simulink model "HMI_C_S_28379D_FW"  (R2024b)
settings: Solver=ode4  StartTime=0.0  StopTime=Inf  FixedStep=Ts  RelTol=1e-3  EnableMultiTasking=on
InitFcn:
  | Ts=1e-4
model workspace (MAT data in the model file):
  encoderResolution = 2000
  hallOffset = '0.5'
  indexOffset = 850
  polePairs = '4'
libraries: simulink x4, c2837xDlib x2, c280xlib x2, c2802xlib x1
(part 1 of 2)
settings Model: ExtModeTrigDuration=8  Creator=matti  LastModifiedBy=Administrator
settings SolverCC: AlgebraicLoopSolver=TrustRegion  AutoInsertRateTranBlk=on
settings DataIOCC: LimitDataPoints=on  SaveFormat=Array  SignalLoggingSaveFormat=ModelDataLogs  SaveOutput=off  SaveTime=off  ReturnWorkspaceOutputs=off
settings OptimizationCC: DefaultUnderspecifiedDataType=single  OptimizeBlockIOStorage=off  BufferReuse=off  GlobalBufferReuse=off  ExpressionFolding=off  ExpressionDepthLimit=2147483647  LocalBlockOutputs=off  InitFltsAndDblsToZero=on  NoFixptDivByZeroProtection=on  EfficientFloat2IntCast=on  EfficientMapNaN2IntZero=off  LifeSpan=Inf  MaxStackSize=1024  OptimizeDataStoreBuffers=off  BusAssignmentInplaceUpdate=off  EfficientTunableParamExpr=on
settings DebuggingCC: ReadBeforeWriteMsg=DisableAll  WriteAfterWriteMsg=DisableAll  WriteAfterReadMsg=DisableAll  CheckSSInitialOutputMsg=off  UnderspecifiedInitializationDetection=Classic  MergeDetectMultiDrivingBlocksExec=none  SignalResolutionControl=TryResolveAllWithWarning  SolverPrmCheckMsg=warning  InheritedTsInSrcMsg=none  MultiTaskDSMMsg=none  MultiTaskCondExecSysMsg=none  TasksWithSamePriorityMsg=none  SigSpecEnsureSampleTimeMsg=none  IntegerOverflowMsg=none  ParameterPrecisionLossMsg=none  FcnCallInpInsideContextMsg=warning  UnconnectedInputMsg=warning  UnconnectedOutputMsg=warning  UnconnectedLineMsg=warning  StateNameClashWarn=warning  SFUnexpectedBacktrackingDiag=warning  SFNoUnconditionalDefaultTransitionDiag=warning  SFExecutionAtInitializationDiag=none  IntegerSaturationMsg=none  ArithmeticOperatorsInVariantConditions=warning
settings HardwareCC: ProdBitPerChar=16  ProdBitPerInt=16  ProdBitPerPointer=32  ProdBitPerSizeT=32  ProdBitPerPtrDiffT=32  ProdLargestAtomicInteger=Integer  ProdLargestAtomicFloat=None  ProdWordSize=16  ProdLongLongMode=on  ProdHWDeviceType=Texas Instruments->C2000  TargetBitPerChar=16  TargetBitPerInt=16  TargetBitPerPointer=16  TargetLargestAtomicInteger=Integer  TargetIntDivRoundTo=Zero  TargetEndianess=LittleEndian  TargetWordSize=16  TargetHWDeviceType=TI C2000  HardwareBoardFeatureSet=SoCBlockset
settings ModelReferenceCC: EnableRefExpFcnMdlSchedulingChecks=on  PropagateSignalLabelsOutOfModel=off
settings SFSimCC: SimUseLocalCustomCode=off  MATLABDynamicMemAlloc=off  CustomCodeUndefinedFunction=UseInterfaceOnly
settings RTWCC: Description=Embedded Coder  SystemTargetFile=ert.tlc  HardwareBoard=TI Delfino F28379D LaunchPad  TemplateMakefile=ert_default_tmf  GenerateReport=on  RTWUseLocalCustomCode=off  Toolchain=Texas Instruments Code Composer Studio (C2000)  IncludeHyperlinkInReport=on  LaunchReport=on  CodeProfilingSaveOptions=MetricsOnly  GenerateTraceInfo=on  GenerateTraceReport=on  GenerateTraceReportSl=on  GenerateTraceReportSf=on  GenerateTraceReportEml=on  GPUComputeCapability=3.5
settings CodeAppCC: IgnoreCustomStorageClasses=off  CustomSymbolStrType=$N$R$M  StateflowObjectComments=on  InternalIdentifier=Classic
settings ERTTargetCC: CodeReplacementLibrary=TI C28x  MultiwordLength=2048  SupportContinuousTime=on  ExtModeTransport=4  ExtModeStaticAlloc=on  ExtModeAutomaticAllocSize=off  ExtModeStaticAllocSize=10000  ExtModeMexFile=ext_xcp  ExtModeIntrfLevel=Level2 - Open  InlinedParameterPlacement=Hierarchical  ConvertIfToSwitch=off  SuppressUnreachableDefaultCases=off  MemSecPackage=tic2000demospkg  MemSecFuncExecute=code_ramfuncs  DynamicArrayContainerType=coder::array
settings ConfigComp: CovMetricSettings=dw  CovSaveCumulativeToWorkspaceVar=on  CovSaveSingleToWorkspaceVar=on  CovExternalEMLEnable=off  CovSFcnEnable=off
settings SimscapeCC: SimscapeNormalizeSystem=off

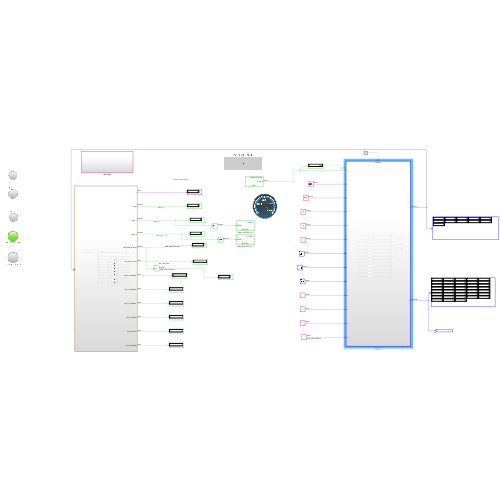
[thumbnail: Simulink's stored preview of the top-level diagram]
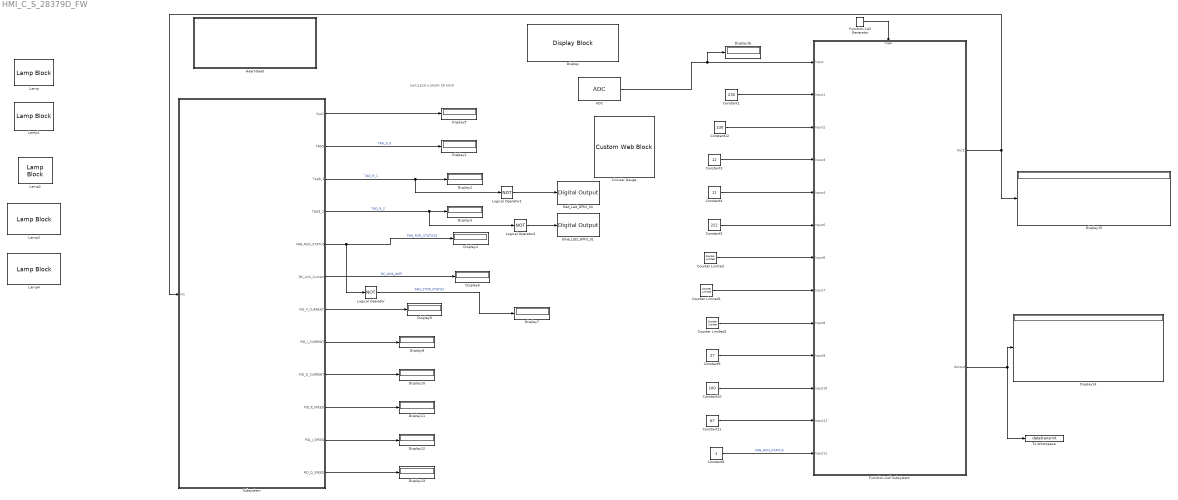
== system HMI_C_S_28379D_FW ==
  note: SHAILESH KUMAR SR MGR
  ADC : c2802xlib/ADC  blkParamProc=C2000_Type4  ADCModule=D  samplingMode=Single sample mode  ADCResolution=12-bit (Single-ended input)  useSOC1=SOC0  useSOC2=SOC0_SOC1  SOCAcquisitionWindow=15  SOCTriggerSource=Software  SOCInterruptTrigger=No ADCINT  Ts=0.001  dType=uint16  postInterrupt=off  interruptSel=ADCINT1  ADCINTContinuous=on  endma=off  chdma=1  conv1=ADCINA0  conv2=ADCINA0 and ADCINB0  conv1_Type4=ADCIN14  conv2_Type4=ADCIN0 and ADCIN1
      settings: LibrarySourceBlock=c2837xDlib/ADC
  Blue_LED_GPIO_31 : c2837xDlib/Digital Output  GPIO_Number=GPIO24~GPIO31  GPIO_Bit0=off  GPIO_BIT0_Toggle=off  GPIO_Bit1=off  GPIO_BIT1_Toggle=off  GPIO_Bit2=off  GPIO_BIT2_Toggle=off  GPIO_Bit3=off  GPIO_BIT3_Toggle=off  GPIO_Bit4=off  GPIO_BIT4_Toggle=off  GPIO_Bit5=off  GPIO_BIT5_Toggle=off  GPIO_Bit6=off  GPIO_BIT6_Toggle=off  GPIO_Bit7=on  GPIO_BIT7_Toggle=off
  Circular Gauge : CustomWebBlock  LabelPosition=Hide  ShowInitialText=on  Configuration="{\"components\":[{\"name\":\"CircularScaleComponent\",\"settings\":{\"bounds\":{\"max\":4096,\"min\":0,\"tickInterval\":\"auto\"},\"direction\":\"cw\",\"flipLimits\":0,\"innerRadius\":0.75,\"internalTickHeightScaleFactor\":1,\"labelColor\":[255,255,200],\"labelFont\":{\"font\":\"Arial\",\"fontSize\":12},\"labelRadius\":0.528,\"labelTransparency\":1,\"minorTickHeightScaleFactor\":0.2,\"needleImage\":{\"size\":[200,50],\"src\":\"data:image\\/svg+xml;base64,PD94bWwgdmVyc2lvbj0iMS4wIiBlbmNvZGluZz0idXRmLTgiPz4KPCEtLSBHZW5lcmF0b3I6IEFkb2JlIElsbHVzdHJhdG9yIDI0LjEuMiwgU1ZHIEV4cG9ydCBQbHVnLUluIC4gU1ZHIFZlcnNpb246IDYuMDAgQnVpbGQgMCkgIC0tPgo8c3ZnIHZlcnNpb249IjEuMSIgaWQ9IkxheWVyXzEiIHhtbG5zPSJodHRwOi8vd3d3LnczLm9yZy8yMDAwL3N2ZyIgeG1sbnM6eGxpbms9Imh0dHA6Ly93d3cudzMub3JnLzE5OTkveGxpbmsiIHg9IjBweCIgeT0iMHB4IgoJIHZpZXdCb3g9IjAgMCAyMDAgNTAiIHN0eWxlPSJlbmFibGUtYmFja2dyb3VuZDpuZXcgMCAwIDIwMCA1MDsiIHhtbDpzcGFjZT0icHJlc2VydmUiPgo8c3R5bGUgdHlwZT0idGV4dC9jc3MiPgoJLnN0MHtmaWxsOiNFQzIxMjc7fQo8L3N0eWxlPgo8cGF0aCBjbGFzcz0ic3QwIiBkPSJNMTYyLjgsMTMuN0MxNjksNC40LDE4MS43LDEuOSwxOTEsOC4xczExLjgsMTguOSw1LjYsMjguMnMtMTguOSwxMS44LTI4LjIsNS42bDAsMAoJQzE1OS4xLDM1LjYsMTU2LjYsMjMsMTYyLjgsMTMuN0wxNjIuOCwxMy43eiBNMTY1LjgsMTUuOGMtNS4xLDcuNi0zLjEsMTcuOSw0LjYsMjNjNy42LDUuMSwxNy45LDMuMSwyMy00LjYKCWM1LjEtNy42LDMuMS0xNy45LTQuNi0yM2wwLDBDMTgxLjIsNi4yLDE3MC45LDguMiwxNjUuOCwxNS44eiIvPgo8cGF0aCBjbGFzcz0ic3QwIiBkPSJNMC40LDI1Ljl2LTMuM2wxNTktMi41Yy0wLjcsMi42LTAuNyw1LjIsMCw3LjhMMC40LDI1Ljl6Ii8+CjxjaXJjbGUgY2xhc3M9InN0MCIgY3g9IjE3OS42IiBjeT0iMjQiIHI9IjAuNyIvPgo8L3N2Zz4K\"},\"needleOffset\":[0.18464878250906522,0],\"needleOrientation\":-45,\"needleRotation\":180,\"needleSize\":{\"height\":0.11741692305346914,\"width\":0.46108337545091255},\"outerRadius\":0.9,\"position\":[0.05,0.05,0.9,0.9],\"referencePoint\":\"auto\",\"scaleAngle\":270,\"scaleAngleOffset\":135,\"scaleColors\":[],\"scaleColorsSize\":0.2,\"scaleDirection\":\"CW\",\"scalePosition\":[0,0,1,1],\"showLabels\":1,\"showMinorTicks\":1,\"showSpanLine\":1,\"showTicks\":1,\"tickColor\":[252,252,197],\"tickTransparency\":1,\"valueBarColor\":[0,114,189],\"valueBarPosition\":[0,0,1,1],\"valueBarSize\":0.2,\"valueBarTransparency\":1}},{\"name\":\"BackgroundImageComponent\",\"settings\":{\"image\":{\"size\":[500,500],\"src\":\"data:image\\/svg+xml;base64,PD94bWwgdmVyc2lvbj0iMS4wIiBlbmNvZGluZz0iVVRGLTgiIHN0YW5kYWxvbmU9Im5vIj8+CjxzdmcKICAgeG1sbnM6ZGM9Imh0dHA6Ly9wdXJsLm9yZy9kYy9lbGVtZW50cy8xLjEvIgogICB4bWxuczpjYz0iaHR0cDovL2NyZWF0aXZlY29tbW9ucy5vcmcvbnMjIgogICB4bWxuczpyZGY9Imh0dHA6Ly93d3cudzMub3JnLzE5OTkvMDIvMjItcmRmLXN5bnRheC1ucyMiCiAgIHhtbG5zOnN2Zz0iaHR0cDovL3d3dy53My5vcmcvMjAwMC9zdmciCiAgIHhtbG5zPSJodHRwOi8vd3d3LnczLm9yZy8yMDAwL3N2ZyIKICAgeG1sbnM6 ...(+9964 chars)\"},\"position\":[0,0,1,1],\"scaleMode\":\"0\"}},{\"name\":\"ForegroundImageComponent\",\"settings\":{\"image\":{\"size\":[0,0],\"src\":\"default\",\"srcOrientation\":[]},\"isForeground\":1,\"position\":[0,0,1,1],\"scaleMode\":\"0\"}}],\"settings\":{\"BindingType\":\"signal\",\"aspectRatio\":1.032258064516129,\"backgroundColor\":[0,0,0,\"1\"],\"backgroundOffset\":1,\"backgroundOpacity\":1,\"direction\":\"cw\",\"fixedAspectRatio\":\"on\",\"flipLimits\":0,\"orientation\":\"horizontal\",\"showBackgroundColor\":false,\"value\":0,\"version\":\"R2023a\"},\"type\":\"CircularGauge\"}"
  Constant1 : Constant  Value=230  OutDataTypeStr=uint16
  Constant10 : Constant  Value=100  OutDataTypeStr=uint16
  Constant11 : Constant  Value=67  OutDataTypeStr=uint16
  Constant12 : Constant  Value=230  OutDataTypeStr=uint16
  Constant3 : Constant  Value=12  OutDataTypeStr=uint16
  Constant4 : Constant  Value=11  OutDataTypeStr=uint16
  Constant5 : Constant  Value=222  OutDataTypeStr=uint16
  Constant6 : Constant  OutDataTypeStr=uint8
  Constant9 : Constant  Value=27  OutDataTypeStr=uint16
  Counter Limited : simulink/Sources/Counter Limited  uplimit=999  tsamp=-1
  Counter Limited1 : simulink/Sources/Counter Limited  uplimit=999  tsamp=-1
  Counter Limited2 : simulink/Sources/Counter Limited  uplimit=999  tsamp=-1
  Display : DisplayBlock  Transparency=1
  Display{1..16} (16 alike) : Display
  Function-Call Generator : simulink/Ports & Subsystems/Function-Call Generator  sample_time=0.1  numberOfIterations=1  DisallowWideOutput=off
  Function-Call Subsystem : Subsystem  TreatAsAtomicUnit=on
  Heart-Beat : Subsystem
  Lamp : LampBlock
  Lamp1 : LampBlock
  Lamp2 : LampBlock
  Lamp3 : LampBlock  LabelPosition=Bottom
  Lamp4 : LampBlock  LabelPosition=Bottom
  Logical Operator : Logic  Operator=NOT  AllPortsSameDT=off  OutDataTypeStr=boolean
  Logical Operator1 : Logic  Operator=NOT  AllPortsSameDT=off  OutDataTypeStr=boolean
  Logical Operator2 : Logic  Operator=NOT  AllPortsSameDT=off  OutDataTypeStr=boolean
  Red_Led_GPIO_34 : c2837xDlib/Digital Output  GPIO_Number=GPIO32~GPIO39  GPIO_Bit0=off  GPIO_BIT0_Toggle=off  GPIO_Bit1=off  GPIO_BIT1_Toggle=off  GPIO_Bit2=on  GPIO_BIT2_Toggle=off  GPIO_Bit3=off  GPIO_BIT3_Toggle=off  GPIO_Bit4=off  GPIO_BIT4_Toggle=off  GPIO_Bit5=off  GPIO_BIT5_Toggle=off  GPIO_Bit6=off  GPIO_BIT6_Toggle=off  GPIO_Bit7=off  GPIO_BIT7_Toggle=off
  Subsystem : Subsystem
  To Workspace : ToWorkspace  VariableName=datatransmit  SampleTime=-1
      settings: Save2DSignal=2-D array (concatenate along first dimension)
  wires:
  Subsystem/12(PID_D_SPEED) -> Display13/1
  Subsystem/1(Out1) -> Display5/1
  Subsystem/5(FAN_RUN_STATUS) -> Display4/1, Logical Operator/1  "FAN_RUN_STATUSS"
  Subsystem/4(TAG9_2) -> Logical Operator2/1, Display3/1  "TAG_9_2"
  Subsystem/3(Tag9_1) -> Logical Operator1/1, Display2/1  "TAG_9_1"
  Subsystem/6(DC_Link_Current) -> Display6/1  "DC_LINK_AMP"
  Subsystem/2(TAG9) -> Display1/1  "TAG_9_0"
  Subsystem/10(PID_P_SPEED) -> Display11/1
  Subsystem/9(PID_D_CURRENT) -> Display10/1
  Subsystem/7(PID_P_CURRENT) -> Display9/1
  Subsystem/8(PID_I_CURRENT) -> Display8/1
  Subsystem/11(PID_I_SPEED) -> Display12/1
  Logical Operator/1 -> Display7/1  "FAN_STOP_STATUS"
  Function-Call Generator/1 -> Function-Call Subsystem/Trigger
  Function-Call Subsystem/1(Out2) -> Subsystem/1(In1), Display15/1
  ADC/1 -> Display16/1, Function-Call Subsystem/1(Input)
  Constant1/1 -> Function-Call Subsystem/2(Input1)
  Constant12/1 -> Function-Call Subsystem/3(Input2)
  Constant3/1 -> Function-Call Subsystem/4(Input3)
  Constant4/1 -> Function-Call Subsystem/5(Input4)
  Constant5/1 -> Function-Call Subsystem/6(Input5)
  Counter Limited/1 -> Function-Call Subsystem/7(Input6)
  Counter Limited1/1 -> Function-Call Subsystem/8(Input7)
  Counter Limited2/1 -> Function-Call Subsystem/9(Input8)
  Constant9/1 -> Function-Call Subsystem/10(Input9)
  Constant10/1 -> Function-Call Subsystem/11(Input10)
  Constant11/1 -> Function-Call Subsystem/12(Input11)
  Constant6/1 -> Function-Call Subsystem/13(Input12)  "FAN_RUN_STATUS"
  Function-Call Subsystem/2(Output) -> To Workspace/1, Display14/1
  Logical Operator1/1 -> Red_Led_GPIO_34/1
  Logical Operator2/1 -> Blue_LED_GPIO_31/1

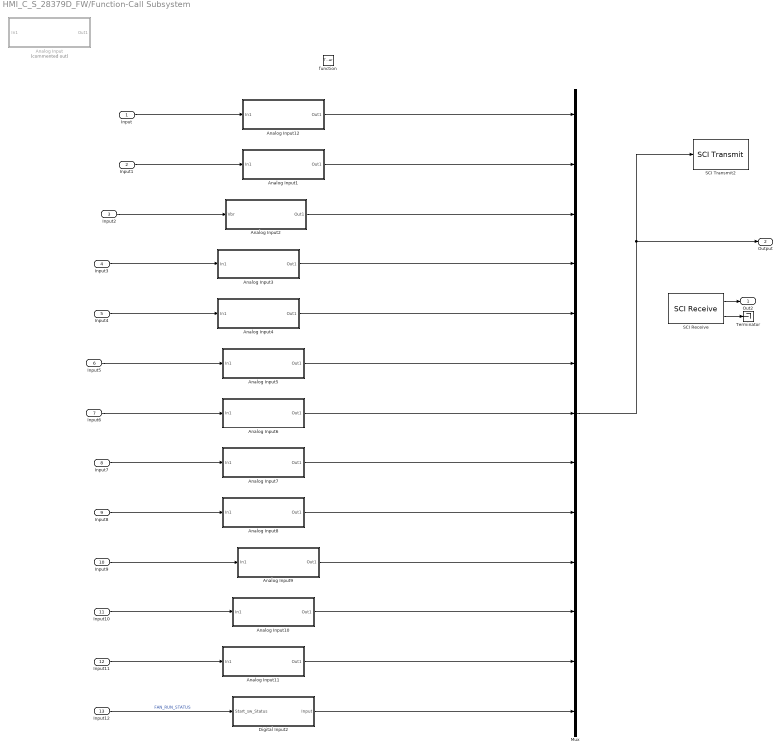
== system HMI_C_S_28379D_FW/Function-Call Subsystem ==
  Input : Inport
  Input1 : Inport  Port=2
  Input2 : Inport  Port=3
  Input3 : Inport  Port=4
  Input4 : Inport  Port=5
  Input5 : Inport  Port=6
  Input6 : Inport  Port=7
  Input7 : Inport  Port=8
  Input8 : Inport  Port=9
  Input9 : Inport  Port=10
  Input10 : Inport  Port=11
  Input11 : Inport  Port=12
  Input12 : Inport  Port=13
  function : TriggerPort  TriggerType=function-call  VariantControl=(inherit)
  Analog Input : Subsystem  Commented=on
  Analog Input1 : Subsystem
  Analog Input10 : Subsystem
  Analog Input11 : Subsystem
  Analog Input12 : Subsystem
  Analog Input2 : Subsystem
  Analog Input3 : Subsystem
  Analog Input4 : Subsystem
  Analog Input5 : Subsystem
  Analog Input6 : Subsystem
  Analog Input7 : Subsystem
  Analog Input8 : Subsystem
  Analog Input9 : Subsystem
  Digital Input2 : Subsystem
  Mux : Mux  Inputs=13
  SCI Receive : c280xlib/SCI Receive  Priority=2  sciModule=B  dataHead='S'  headerCheckMaxCount=16  dataTail='E'  dataType=uint8  dataLenOptions=Length via dialog  dataDim=11  maxDataLength=1  initValue=0  errOption=Output the last received value  errValue=0  sampleTime=-1  blockingMode=off  timeOut=inf  outputStatus=on
      settings: LibrarySourceBlock=c2837xDlib/SCI Receive
  SCI Transmit2 : c280xlib/SCI Transmit  sciModule=B  dataHead='S'  dataTail='E'  frameSize=[1 38]  blockingMode=on  outputStatus=off
      settings: LibrarySourceBlock=c2837xDlib/SCI Transmit
  Terminator : Terminator
  Out2 : Outport
  Output : Outport  Port=2
  wires:
  SCI Receive/1 -> Out2/1
  SCI Receive/2 -> Terminator/1
  Analog Input1/1(Out1) -> Mux/2
  Analog Input2/1(Out1) -> Mux/3
  Analog Input9/1(Out1) -> Mux/10
  Analog Input7/1(Out1) -> Mux/8
  Analog Input4/1(Out1) -> Mux/5
  Analog Input5/1(Out1) -> Mux/6
  Digital Input2/1(Input) -> Mux/13
  Analog Input8/1(Out1) -> Mux/9
  Analog Input10/1(Out1) -> Mux/11
  Analog Input11/1(Out1) -> Mux/12
  Analog Input12/1(Out1) -> Mux/1
  Input1/1 -> Analog Input1/1(In1)
  Input2/1 -> Analog Input2/1(Vbr)
  Input/1 -> Analog Input12/1(In1)
  Input9/1 -> Analog Input9/1(In1)
  Input12/1 -> Digital Input2/1(Start_sw_Status)  "FAN_RUN_STATUS"
  Analog Input3/1(Out1) -> Mux/4
  Input11/1 -> Analog Input11/1(In1)
  Analog Input6/1(Out1) -> Mux/7
  Input10/1 -> Analog Input10/1(In1)
  Mux/1 -> SCI Transmit2/1, Output/1
  Input3/1 -> Analog Input3/1(In1)
  Input4/1 -> Analog Input4/1(In1)
  Input5/1 -> Analog Input5/1(In1)
  Input6/1 -> Analog Input6/1(In1)
  Input7/1 -> Analog Input7/1(In1)
  Input8/1 -> Analog Input8/1(In1)

== system HMI_C_S_28379D_FW/Heart-Beat ==

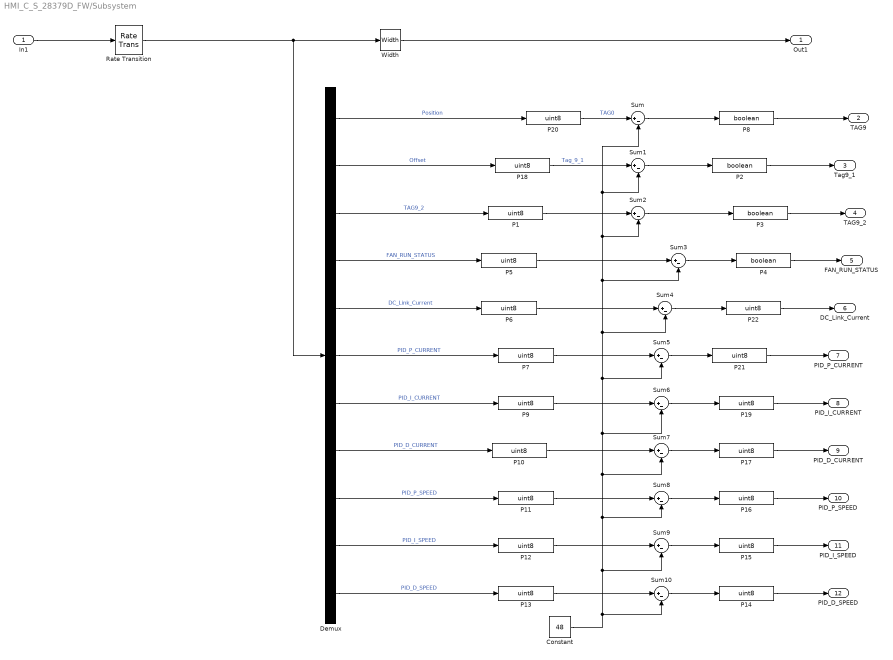
== system HMI_C_S_28379D_FW/Subsystem ==
  In1 : Inport
  Constant : Constant  Value=48  OutDataTypeStr=uint8
  Demux : Demux  Outputs=11
  P{1,5..7,9..22} (18 alike) : DataTypeConversion  OutDataTypeStr=uint8  SaturateOnIntegerOverflow=off  RndMeth=Floor
  P{2..4,8} (4 alike) : DataTypeConversion  OutDataTypeStr=boolean  SaturateOnIntegerOverflow=off  RndMeth=Floor
  Rate Transition : RateTransition
  Sum{,1..10} (11 alike) : Sum  Inputs=|+-
  Width : Width  DataType=uint8
  Out1 : Outport
  TAG9 : Outport  Port=2
  Tag9_1 : Outport  Port=3
  TAG9_2 : Outport  Port=4
  FAN_RUN_STATUS : Outport  Port=5
  DC_Link_Current : Outport  Port=6
  PID_P_CURRENT : Outport  Port=7
  PID_I_CURRENT : Outport  Port=8
  PID_D_CURRENT : Outport  Port=9
  PID_P_SPEED : Outport  Port=10
  PID_I_SPEED : Outport  Port=11
  PID_D_SPEED : Outport  Port=12
  wires:
  Demux/2 -> P18/1  "Offset"
  Demux/1 -> P20/1  "Position"
  Width/1 -> Out1/1
  In1/1 -> Rate Transition/1
  P20/1 -> Sum/1  "TAG0"
  Sum/1 -> P8/1
  P18/1 -> Sum1/1  "Tag_9_1"
  Sum1/1 -> P2/1
  Demux/3 -> P1/1  "TAG9_2"
  Sum2/1 -> P3/1
  Demux/4 -> P5/1  "FAN_RUN_STATUS"
  Sum3/1 -> P4/1
  Demux/5 -> P6/1  "DC_Link_Current"
  Sum4/1 -> P22/1
  Demux/6 -> P7/1  "PID_P_CURRENT"
  Sum5/1 -> P21/1
  Demux/7 -> P9/1  "PID_I_CURRENT"
  Sum6/1 -> P19/1
  Demux/8 -> P10/1  "PID_D_CURRENT"
  Sum7/1 -> P17/1
  Demux/9 -> P11/1  "PID_P_SPEED"
  Sum8/1 -> P16/1
  Demux/10 -> P12/1  "PID_I_SPEED"
  Sum9/1 -> P15/1
  Demux/11 -> P13/1  "PID_D_SPEED"
  Constant/1 -> Sum10/2, Sum9/2, Sum8/2, Sum7/2, Sum6/2, Sum5/2, Sum4/2, Sum3/2, Sum2/2, Sum1/2, Sum/2
  Sum10/1 -> P14/1
  P8/1 -> TAG9/1
  P1/1 -> Sum2/1
  P2/1 -> Tag9_1/1
  P3/1 -> TAG9_2/1
  P4/1 -> FAN_RUN_STATUS/1
  P5/1 -> Sum3/1
  P6/1 -> Sum4/1
  P7/1 -> Sum5/1
  P9/1 -> Sum6/1
  P10/1 -> Sum7/1
  P11/1 -> Sum8/1
  P12/1 -> Sum9/1
  P13/1 -> Sum10/1
  Rate Transition/1 -> Demux/1, Width/1
  P14/1 -> PID_D_SPEED/1
  P15/1 -> PID_I_SPEED/1
  P16/1 -> PID_P_SPEED/1
  P17/1 -> PID_D_CURRENT/1
  P19/1 -> PID_I_CURRENT/1
  P21/1 -> PID_P_CURRENT/1
  P22/1 -> DC_Link_Current/1

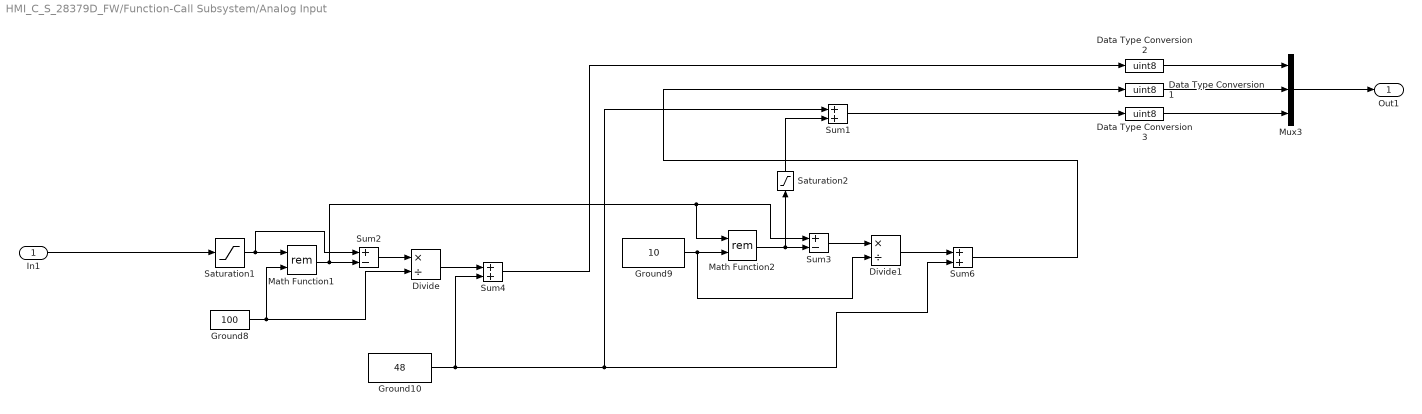
== system HMI_C_S_28379D_FW/Function-Call Subsystem/Analog Input ==
  In1 : Inport
  Data Type Conversion1 : DataTypeConversion  OutDataTypeStr=uint8  SaturateOnIntegerOverflow=off  RndMeth=Floor
  Data Type Conversion2 : DataTypeConversion  OutDataTypeStr=uint8  SaturateOnIntegerOverflow=off  RndMeth=Floor
  Data Type Conversion3 : DataTypeConversion  OutDataTypeStr=uint8  SaturateOnIntegerOverflow=off  RndMeth=Floor
  Divide : Product  Inputs=*/  OutDataTypeStr=int16
  Divide1 : Product  Inputs=*/  OutDataTypeStr=int16
  Ground10 : Constant  Value=48  OutDataTypeStr=int16
  Ground8 : Constant  Value=100  OutDataTypeStr=int16
  Ground9 : Constant  Value=10  OutDataTypeStr=int16
  Math Function1 : Math  Operator=rem  SignedPower=on
  Math Function2 : Math  Operator=rem  SignedPower=on
  Mux3 : Mux  Inputs=3
  Saturation1 : Saturate  UpperLimit=999  LowerLimit=0  OutDataTypeStr=int16
  Saturation2 : Saturate  UpperLimit=9  LowerLimit=0
  Sum1 : Sum  OutDataTypeStr=uint8
  Sum2 : Sum  Inputs=+-  OutDataTypeStr=double
  Sum3 : Sum  Inputs=+-
  Sum4 : Sum  OutDataTypeStr=uint8
  Sum6 : Sum  OutDataTypeStr=uint8
  Out1 : Outport
  wires:
  Saturation1/1 -> Sum2/1, Math Function1/1
  Ground8/1 -> Divide/2, Math Function1/2
  Sum4/1 -> Data Type Conversion2/1
  Sum1/1 -> Data Type Conversion3/1
  Divide/1 -> Sum4/1
  Divide1/1 -> Sum6/1
  Sum2/1 -> Divide/1
  In1/1 -> Saturation1/1
  Data Type Conversion2/1 -> Mux3/1
  Mux3/1 -> Out1/1
  Data Type Conversion3/1 -> Mux3/3
  Data Type Conversion1/1 -> Mux3/2
  Math Function1/1 -> Sum2/2, Math Function2/1, Sum3/1
  Sum3/1 -> Divide1/1
  Sum6/1 -> Data Type Conversion1/1
  Ground10/1 -> Sum4/2, Sum6/2, Sum1/1
  Ground9/1 -> Divide1/2, Math Function2/2
  Math Function2/1 -> Sum3/2, Saturation2/1
  Saturation2/1 -> Sum1/2

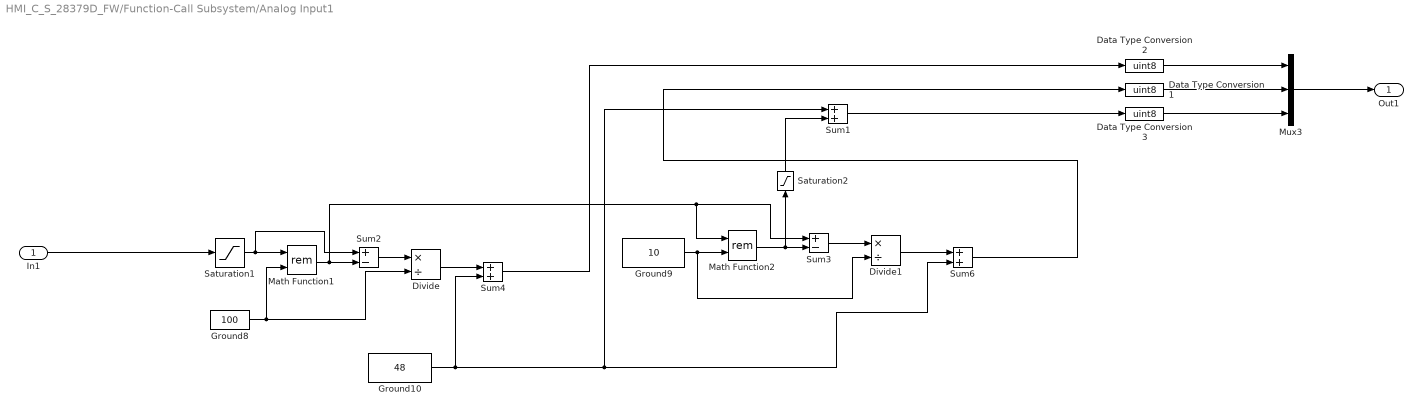
== system HMI_C_S_28379D_FW/Function-Call Subsystem/Analog Input1 ==
  In1 : Inport
  Data Type Conversion1 : DataTypeConversion  OutDataTypeStr=uint8  SaturateOnIntegerOverflow=off  RndMeth=Floor
  Data Type Conversion2 : DataTypeConversion  OutDataTypeStr=uint8  SaturateOnIntegerOverflow=off  RndMeth=Floor
  Data Type Conversion3 : DataTypeConversion  OutDataTypeStr=uint8  SaturateOnIntegerOverflow=off  RndMeth=Floor
  Divide : Product  Inputs=*/  OutDataTypeStr=int16
  Divide1 : Product  Inputs=*/  OutDataTypeStr=int16
  Ground10 : Constant  Value=48  OutDataTypeStr=int16
  Ground8 : Constant  Value=100  OutDataTypeStr=int16
  Ground9 : Constant  Value=10  OutDataTypeStr=int16
  Math Function1 : Math  Operator=rem  SignedPower=on
  Math Function2 : Math  Operator=rem  SignedPower=on
  Mux3 : Mux  Inputs=3
  Saturation1 : Saturate  UpperLimit=999  LowerLimit=0  OutDataTypeStr=int16
  Saturation2 : Saturate  UpperLimit=9  LowerLimit=0
  Sum1 : Sum  OutDataTypeStr=uint8
  Sum2 : Sum  Inputs=+-  OutDataTypeStr=double
  Sum3 : Sum  Inputs=+-
  Sum4 : Sum  OutDataTypeStr=uint8
  Sum6 : Sum  OutDataTypeStr=uint8
  Out1 : Outport
  wires:
  Saturation1/1 -> Sum2/1, Math Function1/1
  Ground8/1 -> Divide/2, Math Function1/2
  Sum4/1 -> Data Type Conversion2/1
  Sum1/1 -> Data Type Conversion3/1
  Divide/1 -> Sum4/1
  Divide1/1 -> Sum6/1
  Sum2/1 -> Divide/1
  In1/1 -> Saturation1/1
  Data Type Conversion2/1 -> Mux3/1
  Mux3/1 -> Out1/1
  Data Type Conversion3/1 -> Mux3/3
  Data Type Conversion1/1 -> Mux3/2
  Math Function1/1 -> Sum2/2, Math Function2/1, Sum3/1
  Sum3/1 -> Divide1/1
  Sum6/1 -> Data Type Conversion1/1
  Ground10/1 -> Sum4/2, Sum6/2, Sum1/1
  Ground9/1 -> Divide1/2, Math Function2/2
  Math Function2/1 -> Sum3/2, Saturation2/1
  Saturation2/1 -> Sum1/2

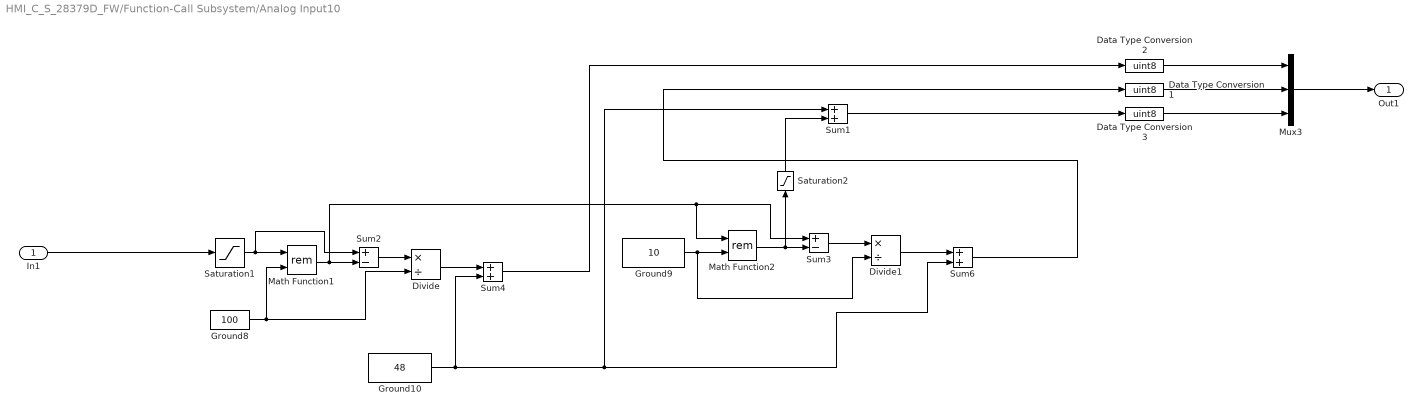
== system HMI_C_S_28379D_FW/Function-Call Subsystem/Analog Input10 ==
  In1 : Inport
  Data Type Conversion1 : DataTypeConversion  OutDataTypeStr=uint8  SaturateOnIntegerOverflow=off  RndMeth=Floor
  Data Type Conversion2 : DataTypeConversion  OutDataTypeStr=uint8  SaturateOnIntegerOverflow=off  RndMeth=Floor
  Data Type Conversion3 : DataTypeConversion  OutDataTypeStr=uint8  SaturateOnIntegerOverflow=off  RndMeth=Floor
  Divide : Product  Inputs=*/  OutDataTypeStr=int16
  Divide1 : Product  Inputs=*/  OutDataTypeStr=int16
  Ground10 : Constant  Value=48  OutDataTypeStr=int16
  Ground8 : Constant  Value=100  OutDataTypeStr=int16
  Ground9 : Constant  Value=10  OutDataTypeStr=int16
  Math Function1 : Math  Operator=rem  SignedPower=on
  Math Function2 : Math  Operator=rem  SignedPower=on
  Mux3 : Mux  Inputs=3
  Saturation1 : Saturate  UpperLimit=999  LowerLimit=0  OutDataTypeStr=int16
  Saturation2 : Saturate  UpperLimit=9  LowerLimit=0
  Sum1 : Sum  OutDataTypeStr=uint8
  Sum2 : Sum  Inputs=+-  OutDataTypeStr=double
  Sum3 : Sum  Inputs=+-
  Sum4 : Sum  OutDataTypeStr=uint8
  Sum6 : Sum  OutDataTypeStr=uint8
  Out1 : Outport
  wires:
  Saturation1/1 -> Sum2/1, Math Function1/1
  Ground8/1 -> Divide/2, Math Function1/2
  Sum4/1 -> Data Type Conversion2/1
  Sum1/1 -> Data Type Conversion3/1
  Divide/1 -> Sum4/1
  Divide1/1 -> Sum6/1
  Sum2/1 -> Divide/1
  In1/1 -> Saturation1/1
  Data Type Conversion2/1 -> Mux3/1
  Mux3/1 -> Out1/1
  Data Type Conversion3/1 -> Mux3/3
  Data Type Conversion1/1 -> Mux3/2
  Math Function1/1 -> Sum2/2, Math Function2/1, Sum3/1
  Sum3/1 -> Divide1/1
  Sum6/1 -> Data Type Conversion1/1
  Ground10/1 -> Sum4/2, Sum6/2, Sum1/1
  Ground9/1 -> Divide1/2, Math Function2/2
  Math Function2/1 -> Sum3/2, Saturation2/1
  Saturation2/1 -> Sum1/2

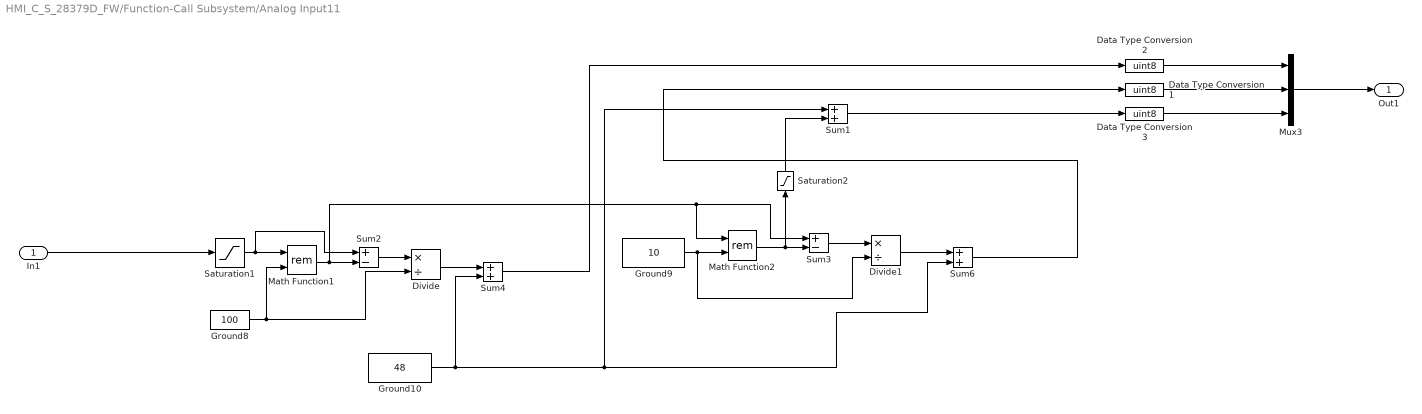
== system HMI_C_S_28379D_FW/Function-Call Subsystem/Analog Input11 ==
  In1 : Inport
  Data Type Conversion1 : DataTypeConversion  OutDataTypeStr=uint8  SaturateOnIntegerOverflow=off  RndMeth=Floor
  Data Type Conversion2 : DataTypeConversion  OutDataTypeStr=uint8  SaturateOnIntegerOverflow=off  RndMeth=Floor
  Data Type Conversion3 : DataTypeConversion  OutDataTypeStr=uint8  SaturateOnIntegerOverflow=off  RndMeth=Floor
  Divide : Product  Inputs=*/  OutDataTypeStr=int16
  Divide1 : Product  Inputs=*/  OutDataTypeStr=int16
  Ground10 : Constant  Value=48  OutDataTypeStr=int16
  Ground8 : Constant  Value=100  OutDataTypeStr=int16
  Ground9 : Constant  Value=10  OutDataTypeStr=int16
  Math Function1 : Math  Operator=rem  SignedPower=on
  Math Function2 : Math  Operator=rem  SignedPower=on
  Mux3 : Mux  Inputs=3
  Saturation1 : Saturate  UpperLimit=999  LowerLimit=0  OutDataTypeStr=int16
  Saturation2 : Saturate  UpperLimit=9  LowerLimit=0
  Sum1 : Sum  OutDataTypeStr=uint8
  Sum2 : Sum  Inputs=+-  OutDataTypeStr=double
  Sum3 : Sum  Inputs=+-
  Sum4 : Sum  OutDataTypeStr=uint8
  Sum6 : Sum  OutDataTypeStr=uint8
  Out1 : Outport
  wires:
  Saturation1/1 -> Sum2/1, Math Function1/1
  Ground8/1 -> Divide/2, Math Function1/2
  Sum4/1 -> Data Type Conversion2/1
  Sum1/1 -> Data Type Conversion3/1
  Divide/1 -> Sum4/1
  Divide1/1 -> Sum6/1
  Sum2/1 -> Divide/1
  In1/1 -> Saturation1/1
  Data Type Conversion2/1 -> Mux3/1
  Mux3/1 -> Out1/1
  Data Type Conversion3/1 -> Mux3/3
  Data Type Conversion1/1 -> Mux3/2
  Math Function1/1 -> Sum2/2, Math Function2/1, Sum3/1
  Sum3/1 -> Divide1/1
  Sum6/1 -> Data Type Conversion1/1
  Ground10/1 -> Sum4/2, Sum6/2, Sum1/1
  Ground9/1 -> Divide1/2, Math Function2/2
  Math Function2/1 -> Sum3/2, Saturation2/1
  Saturation2/1 -> Sum1/2

== system HMI_C_S_28379D_FW/Function-Call Subsystem/Analog Input12 ==
  In1 : Inport
  Subsystem : Subsystem
  Out1 : Outport
  wires:
  Subsystem/1(Out1) -> Out1/1
  In1/1 -> Subsystem/1(In1)

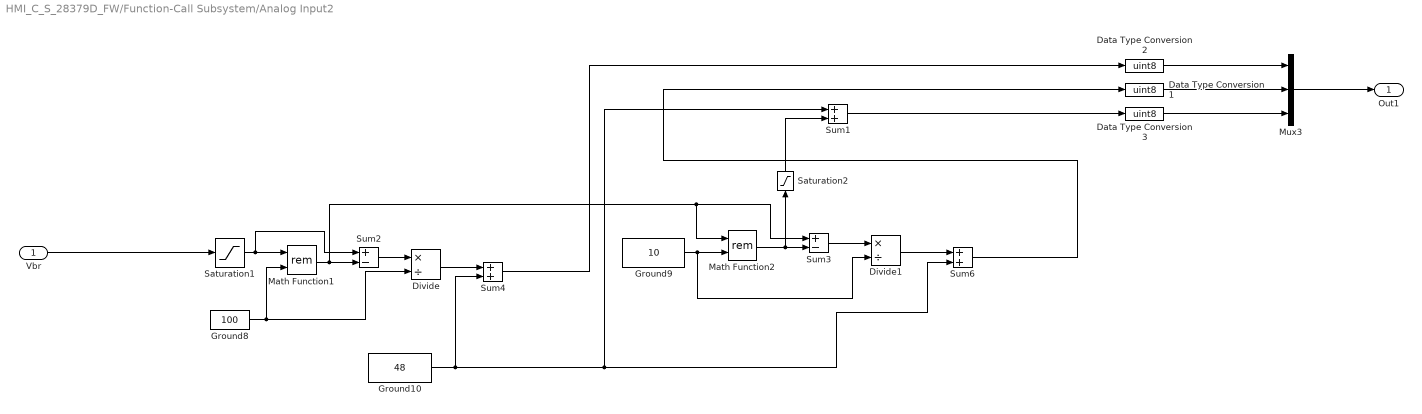
== system HMI_C_S_28379D_FW/Function-Call Subsystem/Analog Input2 ==
  Vbr : Inport
  Data Type Conversion1 : DataTypeConversion  OutDataTypeStr=uint8  SaturateOnIntegerOverflow=off  RndMeth=Floor
  Data Type Conversion2 : DataTypeConversion  OutDataTypeStr=uint8  SaturateOnIntegerOverflow=off  RndMeth=Floor
  Data Type Conversion3 : DataTypeConversion  OutDataTypeStr=uint8  SaturateOnIntegerOverflow=off  RndMeth=Floor
  Divide : Product  Inputs=*/  OutDataTypeStr=int16
  Divide1 : Product  Inputs=*/  OutDataTypeStr=int16
  Ground10 : Constant  Value=48  OutDataTypeStr=int16
  Ground8 : Constant  Value=100  OutDataTypeStr=int16
  Ground9 : Constant  Value=10  OutDataTypeStr=int16
  Math Function1 : Math  Operator=rem  SignedPower=on
  Math Function2 : Math  Operator=rem  SignedPower=on
  Mux3 : Mux  Inputs=3
  Saturation1 : Saturate  UpperLimit=999  LowerLimit=0  OutDataTypeStr=int16
  Saturation2 : Saturate  UpperLimit=9  LowerLimit=0
  Sum1 : Sum  OutDataTypeStr=uint8
  Sum2 : Sum  Inputs=+-  OutDataTypeStr=double
  Sum3 : Sum  Inputs=+-
  Sum4 : Sum  OutDataTypeStr=uint8
  Sum6 : Sum  OutDataTypeStr=uint8
  Out1 : Outport
  wires:
  Saturation1/1 -> Sum2/1, Math Function1/1
  Ground8/1 -> Divide/2, Math Function1/2
  Sum4/1 -> Data Type Conversion2/1
  Sum1/1 -> Data Type Conversion3/1
  Divide/1 -> Sum4/1
  Divide1/1 -> Sum6/1
  Sum2/1 -> Divide/1
  Vbr/1 -> Saturation1/1
  Data Type Conversion2/1 -> Mux3/1
  Mux3/1 -> Out1/1
  Data Type Conversion3/1 -> Mux3/3
  Data Type Conversion1/1 -> Mux3/2
  Math Function1/1 -> Sum2/2, Math Function2/1, Sum3/1
  Sum3/1 -> Divide1/1
  Sum6/1 -> Data Type Conversion1/1
  Ground10/1 -> Sum4/2, Sum6/2, Sum1/1
  Ground9/1 -> Divide1/2, Math Function2/2
  Math Function2/1 -> Sum3/2, Saturation2/1
  Saturation2/1 -> Sum1/2

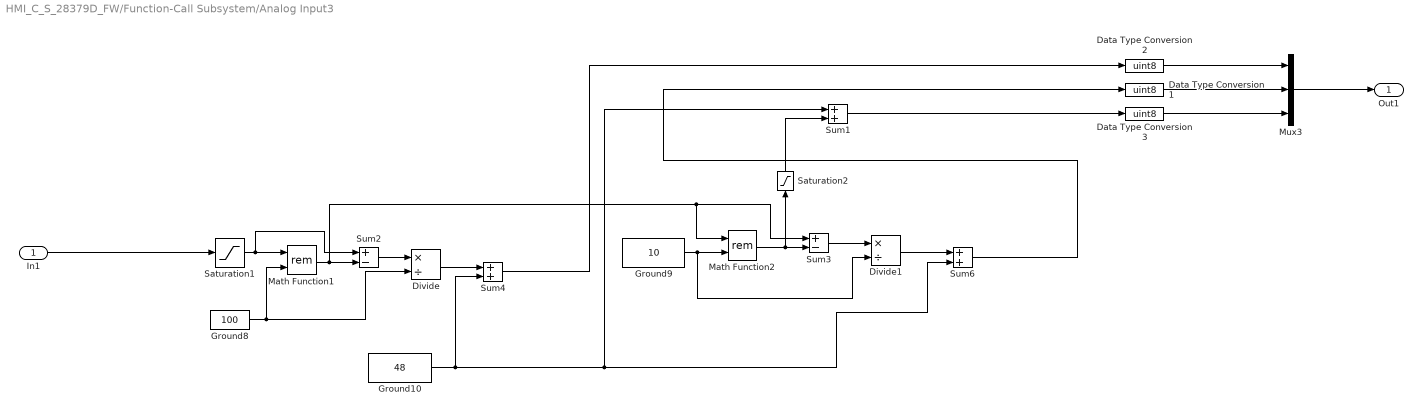
== system HMI_C_S_28379D_FW/Function-Call Subsystem/Analog Input3 ==
  In1 : Inport
  Data Type Conversion1 : DataTypeConversion  OutDataTypeStr=uint8  SaturateOnIntegerOverflow=off  RndMeth=Floor
  Data Type Conversion2 : DataTypeConversion  OutDataTypeStr=uint8  SaturateOnIntegerOverflow=off  RndMeth=Floor
  Data Type Conversion3 : DataTypeConversion  OutDataTypeStr=uint8  SaturateOnIntegerOverflow=off  RndMeth=Floor
  Divide : Product  Inputs=*/  OutDataTypeStr=int16
  Divide1 : Product  Inputs=*/  OutDataTypeStr=int16
  Ground10 : Constant  Value=48  OutDataTypeStr=int16
  Ground8 : Constant  Value=100  OutDataTypeStr=int16
  Ground9 : Constant  Value=10  OutDataTypeStr=int16
  Math Function1 : Math  Operator=rem  SignedPower=on
  Math Function2 : Math  Operator=rem  SignedPower=on
  Mux3 : Mux  Inputs=3
  Saturation1 : Saturate  UpperLimit=999  LowerLimit=0  OutDataTypeStr=int16
  Saturation2 : Saturate  UpperLimit=9  LowerLimit=0
  Sum1 : Sum  OutDataTypeStr=uint8
  Sum2 : Sum  Inputs=+-  OutDataTypeStr=double
  Sum3 : Sum  Inputs=+-
  Sum4 : Sum  OutDataTypeStr=uint8
  Sum6 : Sum  OutDataTypeStr=uint8
  Out1 : Outport
  wires:
  Saturation1/1 -> Sum2/1, Math Function1/1
  Ground8/1 -> Divide/2, Math Function1/2
  Sum4/1 -> Data Type Conversion2/1
  Sum1/1 -> Data Type Conversion3/1
  Divide/1 -> Sum4/1
  Divide1/1 -> Sum6/1
  Sum2/1 -> Divide/1
  In1/1 -> Saturation1/1
  Data Type Conversion2/1 -> Mux3/1
  Mux3/1 -> Out1/1
  Data Type Conversion3/1 -> Mux3/3
  Data Type Conversion1/1 -> Mux3/2
  Math Function1/1 -> Sum2/2, Math Function2/1, Sum3/1
  Sum3/1 -> Divide1/1
  Sum6/1 -> Data Type Conversion1/1
  Ground10/1 -> Sum4/2, Sum6/2, Sum1/1
  Ground9/1 -> Divide1/2, Math Function2/2
  Math Function2/1 -> Sum3/2, Saturation2/1
  Saturation2/1 -> Sum1/2

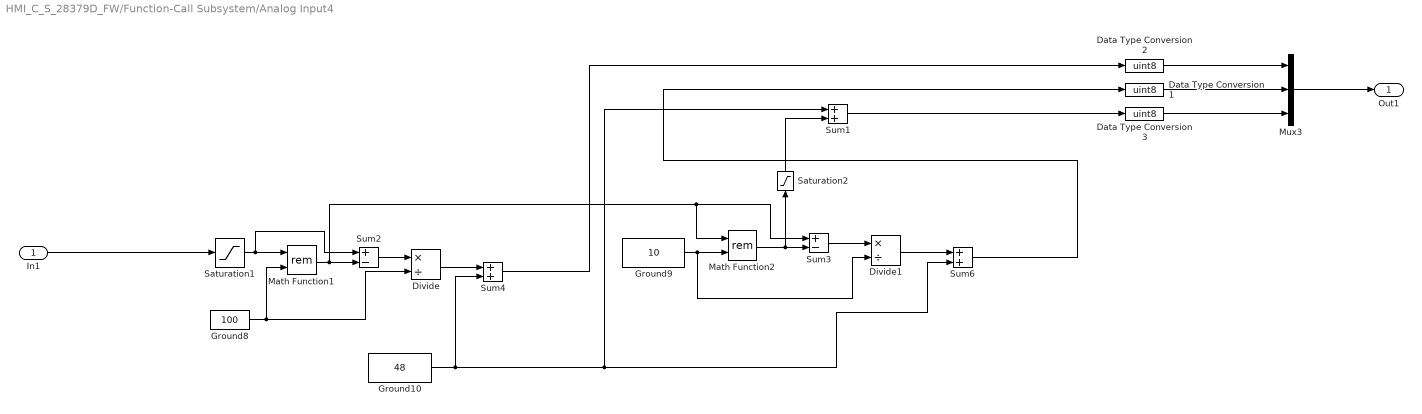
== system HMI_C_S_28379D_FW/Function-Call Subsystem/Analog Input4 ==
  In1 : Inport
  Data Type Conversion1 : DataTypeConversion  OutDataTypeStr=uint8  SaturateOnIntegerOverflow=off  RndMeth=Floor
  Data Type Conversion2 : DataTypeConversion  OutDataTypeStr=uint8  SaturateOnIntegerOverflow=off  RndMeth=Floor
  Data Type Conversion3 : DataTypeConversion  OutDataTypeStr=uint8  SaturateOnIntegerOverflow=off  RndMeth=Floor
  Divide : Product  Inputs=*/  OutDataTypeStr=int16
  Divide1 : Product  Inputs=*/  OutDataTypeStr=int16
  Ground10 : Constant  Value=48  OutDataTypeStr=int16
  Ground8 : Constant  Value=100  OutDataTypeStr=int16
  Ground9 : Constant  Value=10  OutDataTypeStr=int16
  Math Function1 : Math  Operator=rem  SignedPower=on
  Math Function2 : Math  Operator=rem  SignedPower=on
  Mux3 : Mux  Inputs=3
  Saturation1 : Saturate  UpperLimit=999  LowerLimit=0  OutDataTypeStr=int16
  Saturation2 : Saturate  UpperLimit=9  LowerLimit=0
  Sum1 : Sum  OutDataTypeStr=uint8
  Sum2 : Sum  Inputs=+-  OutDataTypeStr=double
  Sum3 : Sum  Inputs=+-
  Sum4 : Sum  OutDataTypeStr=uint8
  Sum6 : Sum  OutDataTypeStr=uint8
  Out1 : Outport
  wires:
  Saturation1/1 -> Sum2/1, Math Function1/1
  Ground8/1 -> Divide/2, Math Function1/2
  Sum4/1 -> Data Type Conversion2/1
  Sum1/1 -> Data Type Conversion3/1
  Divide/1 -> Sum4/1
  Divide1/1 -> Sum6/1
  Sum2/1 -> Divide/1
  In1/1 -> Saturation1/1
  Data Type Conversion2/1 -> Mux3/1
  Mux3/1 -> Out1/1
  Data Type Conversion3/1 -> Mux3/3
  Data Type Conversion1/1 -> Mux3/2
  Math Function1/1 -> Sum2/2, Math Function2/1, Sum3/1
  Sum3/1 -> Divide1/1
  Sum6/1 -> Data Type Conversion1/1
  Ground10/1 -> Sum4/2, Sum6/2, Sum1/1
  Ground9/1 -> Divide1/2, Math Function2/2
  Math Function2/1 -> Sum3/2, Saturation2/1
  Saturation2/1 -> Sum1/2

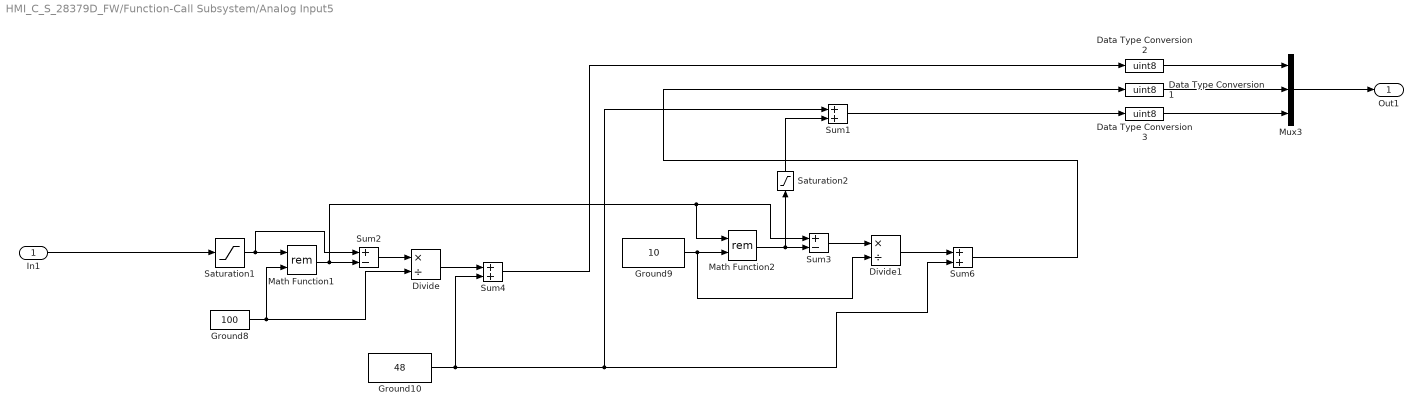
== system HMI_C_S_28379D_FW/Function-Call Subsystem/Analog Input5 ==
  In1 : Inport
  Data Type Conversion1 : DataTypeConversion  OutDataTypeStr=uint8  SaturateOnIntegerOverflow=off  RndMeth=Floor
  Data Type Conversion2 : DataTypeConversion  OutDataTypeStr=uint8  SaturateOnIntegerOverflow=off  RndMeth=Floor
  Data Type Conversion3 : DataTypeConversion  OutDataTypeStr=uint8  SaturateOnIntegerOverflow=off  RndMeth=Floor
  Divide : Product  Inputs=*/  OutDataTypeStr=int16
  Divide1 : Product  Inputs=*/  OutDataTypeStr=int16
  Ground10 : Constant  Value=48  OutDataTypeStr=int16
  Ground8 : Constant  Value=100  OutDataTypeStr=int16
  Ground9 : Constant  Value=10  OutDataTypeStr=int16
  Math Function1 : Math  Operator=rem  SignedPower=on
  Math Function2 : Math  Operator=rem  SignedPower=on
  Mux3 : Mux  Inputs=3
  Saturation1 : Saturate  UpperLimit=999  LowerLimit=0  OutDataTypeStr=int16
  Saturation2 : Saturate  UpperLimit=9  LowerLimit=0
  Sum1 : Sum  OutDataTypeStr=uint8
  Sum2 : Sum  Inputs=+-  OutDataTypeStr=double
  Sum3 : Sum  Inputs=+-
  Sum4 : Sum  OutDataTypeStr=uint8
  Sum6 : Sum  OutDataTypeStr=uint8
  Out1 : Outport
  wires:
  Saturation1/1 -> Sum2/1, Math Function1/1
  Ground8/1 -> Divide/2, Math Function1/2
  Sum4/1 -> Data Type Conversion2/1
  Sum1/1 -> Data Type Conversion3/1
  Divide/1 -> Sum4/1
  Divide1/1 -> Sum6/1
  Sum2/1 -> Divide/1
  In1/1 -> Saturation1/1
  Data Type Conversion2/1 -> Mux3/1
  Mux3/1 -> Out1/1
  Data Type Conversion3/1 -> Mux3/3
  Data Type Conversion1/1 -> Mux3/2
  Math Function1/1 -> Sum2/2, Math Function2/1, Sum3/1
  Sum3/1 -> Divide1/1
  Sum6/1 -> Data Type Conversion1/1
  Ground10/1 -> Sum4/2, Sum6/2, Sum1/1
  Ground9/1 -> Divide1/2, Math Function2/2
  Math Function2/1 -> Sum3/2, Saturation2/1
  Saturation2/1 -> Sum1/2

== system HMI_C_S_28379D_FW/Function-Call Subsystem/Analog Input6 ==
  In1 : Inport
  Data Type Conversion1 : DataTypeConversion  OutDataTypeStr=uint8  SaturateOnIntegerOverflow=off  RndMeth=Floor
  Data Type Conversion2 : DataTypeConversion  OutDataTypeStr=uint8  SaturateOnIntegerOverflow=off  RndMeth=Floor
  Data Type Conversion3 : DataTypeConversion  OutDataTypeStr=uint8  SaturateOnIntegerOverflow=off  RndMeth=Floor
  Divide : Product  Inputs=*/  OutDataTypeStr=int16
  Divide1 : Product  Inputs=*/  OutDataTypeStr=int16
  Ground10 : Constant  Value=48  OutDataTypeStr=int16
  Ground8 : Constant  Value=100  OutDataTypeStr=int16
  Ground9 : Constant  Value=10  OutDataTypeStr=int16
  Math Function1 : Math  Operator=rem  SignedPower=on
  Math Function2 : Math  Operator=rem  SignedPower=on
  Mux3 : Mux  Inputs=3
  Saturation1 : Saturate  UpperLimit=999  LowerLimit=0  OutDataTypeStr=int16
  Saturation2 : Saturate  UpperLimit=9  LowerLimit=0
  Sum1 : Sum  OutDataTypeStr=uint8
  Sum2 : Sum  Inputs=+-  OutDataTypeStr=double
  Sum3 : Sum  Inputs=+-
  Sum4 : Sum  OutDataTypeStr=uint8
  Sum6 : Sum  OutDataTypeStr=uint8
  Out1 : Outport
  wires:
  Saturation1/1 -> Sum2/1, Math Function1/1
  Ground8/1 -> Divide/2, Math Function1/2
  Sum4/1 -> Data Type Conversion2/1
  Sum1/1 -> Data Type Conversion3/1
  Divide/1 -> Sum4/1
  Divide1/1 -> Sum6/1
  Sum2/1 -> Divide/1
  In1/1 -> Saturation1/1
  Data Type Conversion2/1 -> Mux3/1
  Mux3/1 -> Out1/1
  Data Type Conversion3/1 -> Mux3/3
  Data Type Conversion1/1 -> Mux3/2
  Math Function1/1 -> Sum2/2, Math Function2/1, Sum3/1
  Sum3/1 -> Divide1/1
  Sum6/1 -> Data Type Conversion1/1
  Ground10/1 -> Sum4/2, Sum6/2, Sum1/1
  Ground9/1 -> Divide1/2, Math Function2/2
  Math Function2/1 -> Sum3/2, Saturation2/1
  Saturation2/1 -> Sum1/2

== system HMI_C_S_28379D_FW/Function-Call Subsystem/Analog Input7 ==
  In1 : Inport
  Data Type Conversion1 : DataTypeConversion  OutDataTypeStr=uint8  SaturateOnIntegerOverflow=off  RndMeth=Floor
  Data Type Conversion2 : DataTypeConversion  OutDataTypeStr=uint8  SaturateOnIntegerOverflow=off  RndMeth=Floor
  Data Type Conversion3 : DataTypeConversion  OutDataTypeStr=uint8  SaturateOnIntegerOverflow=off  RndMeth=Floor
  Divide : Product  Inputs=*/  OutDataTypeStr=int16
  Divide1 : Product  Inputs=*/  OutDataTypeStr=int16
  Ground10 : Constant  Value=48  OutDataTypeStr=int16
  Ground8 : Constant  Value=100  OutDataTypeStr=int16
  Ground9 : Constant  Value=10  OutDataTypeStr=int16
  Math Function1 : Math  Operator=rem  SignedPower=on
  Math Function2 : Math  Operator=rem  SignedPower=on
  Mux3 : Mux  Inputs=3
  Saturation1 : Saturate  UpperLimit=999  LowerLimit=0  OutDataTypeStr=int16
  Saturation2 : Saturate  UpperLimit=9  LowerLimit=0
  Sum1 : Sum  OutDataTypeStr=uint8
  Sum2 : Sum  Inputs=+-  OutDataTypeStr=double
  Sum3 : Sum  Inputs=+-
  Sum4 : Sum  OutDataTypeStr=uint8
  Sum6 : Sum  OutDataTypeStr=uint8
  Out1 : Outport
  wires:
  Saturation1/1 -> Sum2/1, Math Function1/1
  Ground8/1 -> Divide/2, Math Function1/2
  Sum4/1 -> Data Type Conversion2/1
  Sum1/1 -> Data Type Conversion3/1
  Divide/1 -> Sum4/1
  Divide1/1 -> Sum6/1
  Sum2/1 -> Divide/1
  In1/1 -> Saturation1/1
  Data Type Conversion2/1 -> Mux3/1
  Mux3/1 -> Out1/1
  Data Type Conversion3/1 -> Mux3/3
  Data Type Conversion1/1 -> Mux3/2
  Math Function1/1 -> Sum2/2, Math Function2/1, Sum3/1
  Sum3/1 -> Divide1/1
  Sum6/1 -> Data Type Conversion1/1
  Ground10/1 -> Sum4/2, Sum6/2, Sum1/1
  Ground9/1 -> Divide1/2, Math Function2/2
  Math Function2/1 -> Sum3/2, Saturation2/1
  Saturation2/1 -> Sum1/2

== system HMI_C_S_28379D_FW/Function-Call Subsystem/Analog Input8 ==
  In1 : Inport
  Data Type Conversion1 : DataTypeConversion  OutDataTypeStr=uint8  SaturateOnIntegerOverflow=off  RndMeth=Floor
  Data Type Conversion2 : DataTypeConversion  OutDataTypeStr=uint8  SaturateOnIntegerOverflow=off  RndMeth=Floor
  Data Type Conversion3 : DataTypeConversion  OutDataTypeStr=uint8  SaturateOnIntegerOverflow=off  RndMeth=Floor
  Divide : Product  Inputs=*/  OutDataTypeStr=int16
  Divide1 : Product  Inputs=*/  OutDataTypeStr=int16
  Ground10 : Constant  Value=48  OutDataTypeStr=int16
  Ground8 : Constant  Value=100  OutDataTypeStr=int16
  Ground9 : Constant  Value=10  OutDataTypeStr=int16
  Math Function1 : Math  Operator=rem  SignedPower=on
  Math Function2 : Math  Operator=rem  SignedPower=on
  Mux3 : Mux  Inputs=3
  Saturation1 : Saturate  UpperLimit=999  LowerLimit=0  OutDataTypeStr=int16
  Saturation2 : Saturate  UpperLimit=9  LowerLimit=0
  Sum1 : Sum  OutDataTypeStr=uint8
  Sum2 : Sum  Inputs=+-  OutDataTypeStr=double
  Sum3 : Sum  Inputs=+-
  Sum4 : Sum  OutDataTypeStr=uint8
  Sum6 : Sum  OutDataTypeStr=uint8
  Out1 : Outport
  wires:
  Saturation1/1 -> Sum2/1, Math Function1/1
  Ground8/1 -> Divide/2, Math Function1/2
  Sum4/1 -> Data Type Conversion2/1
  Sum1/1 -> Data Type Conversion3/1
  Divide/1 -> Sum4/1
  Divide1/1 -> Sum6/1
  Sum2/1 -> Divide/1
  In1/1 -> Saturation1/1
  Data Type Conversion2/1 -> Mux3/1
  Mux3/1 -> Out1/1
  Data Type Conversion3/1 -> Mux3/3
  Data Type Conversion1/1 -> Mux3/2
  Math Function1/1 -> Sum2/2, Math Function2/1, Sum3/1
  Sum3/1 -> Divide1/1
  Sum6/1 -> Data Type Conversion1/1
  Ground10/1 -> Sum4/2, Sum6/2, Sum1/1
  Ground9/1 -> Divide1/2, Math Function2/2
  Math Function2/1 -> Sum3/2, Saturation2/1
  Saturation2/1 -> Sum1/2

== system HMI_C_S_28379D_FW/Function-Call Subsystem/Analog Input9 ==
  In1 : Inport
  Data Type Conversion1 : DataTypeConversion  OutDataTypeStr=uint8  SaturateOnIntegerOverflow=off  RndMeth=Floor
  Data Type Conversion2 : DataTypeConversion  OutDataTypeStr=uint8  SaturateOnIntegerOverflow=off  RndMeth=Floor
  Data Type Conversion3 : DataTypeConversion  OutDataTypeStr=uint8  SaturateOnIntegerOverflow=off  RndMeth=Floor
  Divide : Product  Inputs=*/  OutDataTypeStr=int16
  Divide1 : Product  Inputs=*/  OutDataTypeStr=int16
  Ground10 : Constant  Value=48  OutDataTypeStr=int16
  Ground8 : Constant  Value=100  OutDataTypeStr=int16
  Ground9 : Constant  Value=10  OutDataTypeStr=int16
  Math Function1 : Math  Operator=rem  SignedPower=on
  Math Function2 : Math  Operator=rem  SignedPower=on
  Mux3 : Mux  Inputs=3
  Saturation1 : Saturate  UpperLimit=999  LowerLimit=0  OutDataTypeStr=int16
  Saturation2 : Saturate  UpperLimit=9  LowerLimit=0
  Sum1 : Sum  OutDataTypeStr=uint8
  Sum2 : Sum  Inputs=+-  OutDataTypeStr=double
  Sum3 : Sum  Inputs=+-
  Sum4 : Sum  OutDataTypeStr=uint8
  Sum6 : Sum  OutDataTypeStr=uint8
  Out1 : Outport
  wires:
  Saturation1/1 -> Sum2/1, Math Function1/1
  Ground8/1 -> Divide/2, Math Function1/2
  Sum4/1 -> Data Type Conversion2/1
  Sum1/1 -> Data Type Conversion3/1
  Divide/1 -> Sum4/1
  Divide1/1 -> Sum6/1
  Sum2/1 -> Divide/1
  In1/1 -> Saturation1/1
  Data Type Conversion2/1 -> Mux3/1
  Mux3/1 -> Out1/1
  Data Type Conversion3/1 -> Mux3/3
  Data Type Conversion1/1 -> Mux3/2
  Math Function1/1 -> Sum2/2, Math Function2/1, Sum3/1
  Sum3/1 -> Divide1/1
  Sum6/1 -> Data Type Conversion1/1
  Ground10/1 -> Sum4/2, Sum6/2, Sum1/1
  Ground9/1 -> Divide1/2, Math Function2/2
  Math Function2/1 -> Sum3/2, Saturation2/1
  Saturation2/1 -> Sum1/2

== system HMI_C_S_28379D_FW/Function-Call Subsystem/Digital Input2 ==
  Start_sw_Status : Inport
  Ground10 : Constant  Value=48  OutDataTypeStr=int16
  Saturation1 : Saturate  UpperLimit=1  LowerLimit=0  OutDataTypeStr=double
  Sum4 : Sum  OutDataTypeStr=uint8
  Input : Outport
  wires:
  Saturation1/1 -> Sum4/1
  Start_sw_Status/1 -> Saturation1/1
  Ground10/1 -> Sum4/2
  Sum4/1 -> Input/1
